simulink model "PodesavanjeRegulatoraGMK"  (R2016a)
settings: Solver=VariableStepAuto  StartTime=0.0  StopTime=50  RelTol=1e-3
settings Model: Creator=M-Pc  LastModifiedBy=M-Pc

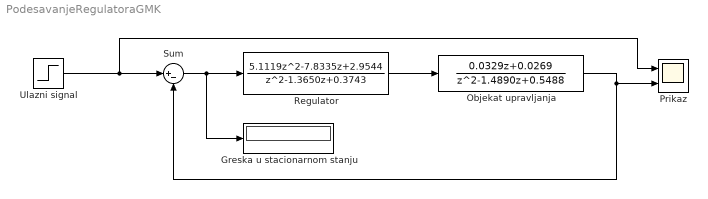
== system PodesavanjeRegulatoraGMK ==
  Greska u stacionarnom stanju : Display
  Objekat upravljanja : DiscreteTransferFcn  Numerator=[0.0329 0.0269]  Denominator=[1 -1.4890 0.5488]  SampleTime=1
  Prikaz : Scope  NumInputPorts=2
  Regulator : DiscreteTransferFcn  Numerator=[5.1119 -7.8335 2.9544]  Denominator=[1 -1.3650 0.3743]  SampleTime=1
  Sum : Sum  Inputs=|+-
  Ulazni signal : Step  SampleTime=0
  wires:
  Ulazni signal/1 -> Prikaz/1, Sum/1
  Sum/1 -> Greska u stacionarnom stanju/1, Regulator/1
  Regulator/1 -> Objekat upravljanja/1
  Objekat upravljanja/1 -> Sum/2, Prikaz/2
